simulink model "Part_1"  (R2020b)
settings: Solver=VariableStepAuto  StartTime=0.0  StopTime=10  RelTol=1e-3
settings Model: Creator=hp  LastModifiedBy=hp
settings DataIOCC: ReturnWorkspaceOutputs=off
settings DebuggingCC: ArithmeticOperatorsInVariantConditions=warning
settings SFSimCC: SimUseLocalCustomCode=off  CustomCodeUndefinedFunction=UseInterfaceOnly
settings RTWCC: RTWUseLocalCustomCode=off

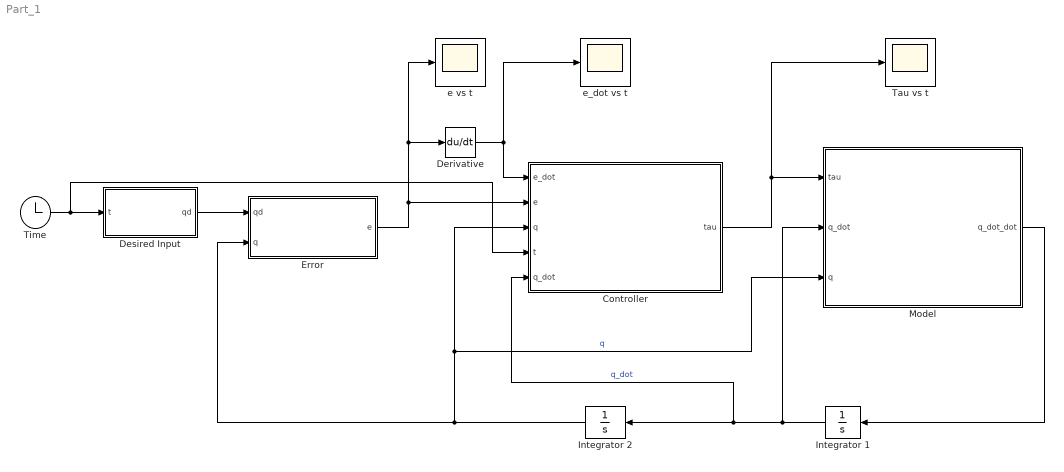
== system Part_1 ==
  Controller : MATLAB Function  TreatAsAtomicUnit=on
  Derivative : Derivative
  Desired Input : MATLAB Function  TreatAsAtomicUnit=on
  Error : MATLAB Function  TreatAsAtomicUnit=on
  Integrator 1 : Integrator  InitialCondition=[0;0]
  Integrator 2 : Integrator  InitialCondition=[0;0]
  Model : MATLAB Function  TreatAsAtomicUnit=on
  Tau vs t : Scope
  Time : Clock
  e vs t : Scope
  e_dot vs t : Scope
  wires:
  Time/1 -> Controller/4(t), Desired Input/1(t)
  Error/1(e) -> Derivative/1, e vs t/1, Controller/2(e)
  Derivative/1 -> Controller/1(e_dot), e_dot vs t/1
  Controller/1(tau) -> Tau vs t/1, Model/1(tau)
  Model/1(q_dot_dot) -> Integrator 1/1
  Integrator 1/1 -> Controller/5(q_dot), Integrator 2/1, Model/2(q_dot)  "q_dot"
  Integrator 2/1 -> Controller/3(q), Model/3(q), Error/2(q)  "q"
  Desired Input/1(qd) -> Error/1(qd)

== matlab function Part_1/Error ==
  data: qd input; q input; e output
function e= fcn(qd,q)

e = q - qd;

end

== matlab function Part_1/Desired Input ==
  data: t input; qd output
function qd = fnc(t)

qd = [ (pi/3)+((pi/6)*sin(t)) ;
      (pi/4)+((pi/6)*cos(t)) ];
  
end

== matlab function Part_1/Controller ==
  data: e_dot input; e input; tau output; q input; t input; q_dot input
function tau= fcn(e_dot,e,q,t,q_dot)

kp = 5;
kd = 5;

m1=3.473; m2=0.196; l1=1; l2=1; g=9.81;
theta1_dot=q_dot(1,1); theta2_dot=q_dot(2,1);
theta1=q(1,1); theta2=q(2,1);
f1=5.3; f2=1.1;

mass_matrix = [ ((m1+m2)*l1*l1)+(m2*l2*l2)+(2*m2*l1*l2*cos(theta2)) , (m2*l2*l2)+(m2*l1*l2*cos(theta2)) ;
                (m2*l2*l2)+(m2*l1*l2*cos(theta2))                   , (m2*l2*l2)                       ];
            
qd_dot = [  (pi*cos(t))/6 ;
           -(pi*sin(t))/6 ];
       
qd_dot_dot = [ -(pi*sin(t))/6 ;
               -(pi*cos(t))/6 ];

friction_term = [ f1, 0 ; f2, 0] * q_dot ; 
              
gravity_term = [ ((m1+m2)*g*l1*cos(theta1))+(m2*g*l2*cos(theta1+theta2)) ;
                  m2*g*l2*cos(theta1+theta2)                            ];
              
Vm = [ -2*m2*l1*l2*theta2_dot*sin(theta2), -m2*l1*l2*theta2_dot*sin(theta2) ;
        m2*l1*l2*theta1_dot*sin(theta2)  , 0                               ];

feed_forward = (gravity_term) + (mass_matrix*qd_dot_dot) + (friction_term) + (Vm*qd_dot) ;
feed_backward = -(kp*e)-(kd*e_dot);

tau = feed_forward + feed_backward;

end

== matlab function Part_1/Model ==
  data: tau input; q_dot_dot output; q_dot input; q input
function q_dot_dot  = fcn(tau,q_dot,q)

m1=3.473; m2=0.196; l1=1; l2=1; g=9.81;
f1=5.3; f2=1.1;

theta1_dot=q_dot(1,1); theta2_dot=q_dot(2,1);
theta1=q(1,1); theta2=q(2,1);

mass_matrix = [ ((m1+m2)*l1*l1)+(m2*l2*l2)+(2*m2*l1*l2*cos(theta2)) , (m2*l2*l2)+(m2*l1*l2*cos(theta2)) ;
                (m2*l2*l2)+(m2*l1*l2*cos(theta2))                   , (m2*l2*l2)                       ];
             
coriolis_term = [ -m2*l1*l2*((2*theta1_dot*theta2_dot)+(theta2_dot*theta2_dot))*sin(theta2) ;
                               m2*l1*l2*theta1_dot*theta1_dot*sin(theta2)                  ];
                           
friction_term = [ f1, 0 ; f2, 0] * q_dot ; 
              
gravity_term = [ ((m1+m2)*g*l1*cos(theta1))+(m2*g*l2*cos(theta1+theta2)) ;
                  m2*g*l2*cos(theta1+theta2)                            ];
              
q_dot_dot = mass_matrix \ (tau-coriolis_term-gravity_term-friction_term);           
                                                                                        
end
